simulink model "WorkstationModel"  (Simulink 7.9)
settings: Solver=VariableStepDiscrete  StartTime=0.0  StopTime=100.0  RelTol=1e-3
undefined symbols (not defined in the file or in its folder): des, gcbh
settings Model: Creator=tsprock3  LastModifiedBy=tsprock3
settings DebuggingCC: SimStateOlderReleaseMsg=warning

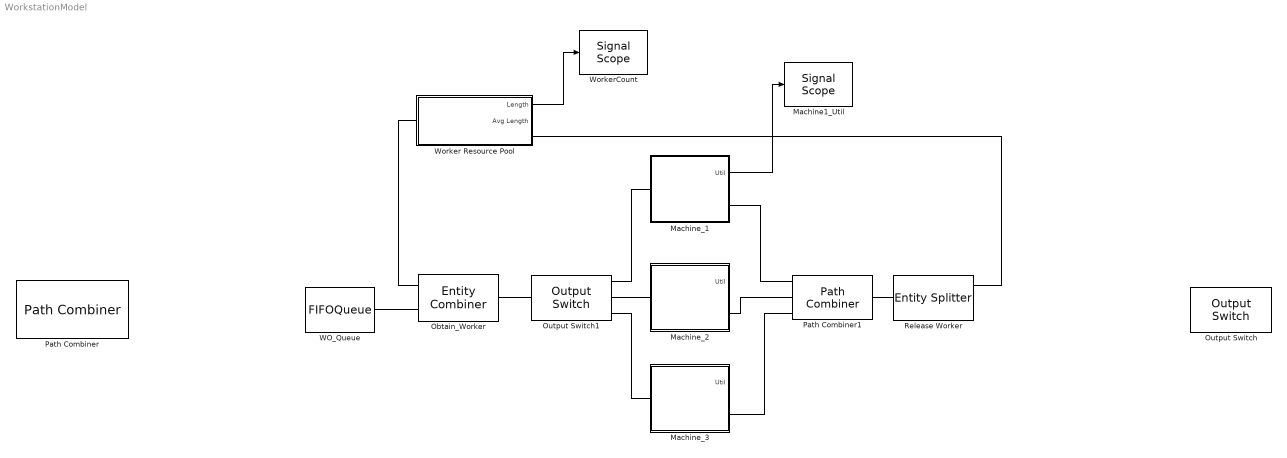
== system WorkstationModel ==
  Machine1_Util : SignalScope  LoadFcn=des.scope.CallbackSupport('seLoadFcn',gcbh)  StartFcn=des.scope.CallbackSupport('seStartFcn',gcbh)  StopFcn=des.scope.CallbackSupport('seStopFcn',gcbh)
      settings: CopyFcn=des.scope.CallbackSupport('seCopyFcn',gcbh)  DeleteFcn=des.scope.CallbackSupport('seDeleteFcn',gcbh)  PreSaveFcn=des.scope.CallbackSupport('sePreSaveFcn',gcbh)  NameChangeFcn=des.scope.CallbackSupport('seNameChangeFcn',gcbh)  OpenFcn=des.scope.CallbackSupport('seOpenFcn',gcbh)
  Machine_1 : Subsystem  mask{mttf=25, mttr=5, ct=3}
      mask prompts: mttf "MTTF (exp)"; mttr "MTTR (exp)"; ct "Process_Time (exp)"
  Machine_2 : Subsystem  mask{mttf=25, mttr=5, ct=3}
      mask prompts: mttf "MTTF (exp)"; mttr "MTTR (exp)"; ct "Process_Time (exp)"
  Machine_3 : Subsystem  mask{mttf=25, mttr=5, ct=3}
      mask prompts: mttf "MTTF (exp)"; mttr "MTTR (exp)"; ct "Process_Time (exp)"
  Obtain_Worker : EntityCombiner  NumberInputPorts=2
  Output Switch : OutputSwitch
  Output Switch1 : OutputSwitch
  Path Combiner : PathCombiner
  Path Combiner1 : PathCombiner
  Release Worker : EntitySplitter  NumberOutputPorts=2
  WO_Queue : FIFOQueue
  Worker Resource Pool : Subsystem  mask{NumberOfEventsPerPeriod=2}
      mask prompts: NumberOfEventsPerPeriod "# of Workers"
  WorkerCount : SignalScope  LoadFcn=des.scope.CallbackSupport('seLoadFcn',gcbh)  StartFcn=des.scope.CallbackSupport('seStartFcn',gcbh)  StopFcn=des.scope.CallbackSupport('seStopFcn',gcbh)
      settings: CopyFcn=des.scope.CallbackSupport('seCopyFcn',gcbh)  DeleteFcn=des.scope.CallbackSupport('seDeleteFcn',gcbh)  PreSaveFcn=des.scope.CallbackSupport('sePreSaveFcn',gcbh)  NameChangeFcn=des.scope.CallbackSupport('seNameChangeFcn',gcbh)  OpenFcn=des.scope.CallbackSupport('seOpenFcn',gcbh)
  wires:
  Worker Resource Pool/1(Length) -> WorkerCount/1
  Machine_1/1(Util) -> Machine1_Util/1
  connections:
  WO_Queue/RConn1 -- Obtain_Worker/LConn2
  Worker Resource Pool/LConn1 -- Obtain_Worker/LConn1
  Obtain_Worker/RConn1 -- Output Switch1/LConn1
  Output Switch1/RConn1 -- Machine_1/LConn1
  Output Switch1/RConn2 -- Machine_2/LConn1
  Output Switch1/RConn3 -- Machine_3/LConn1
  Machine_2/RConn1 -- Path Combiner1/LConn2
  Machine_1/RConn1 -- Path Combiner1/LConn1
  Machine_3/RConn1 -- Path Combiner1/LConn3
  Path Combiner1/RConn1 -- Release Worker/LConn1
  Release Worker/RConn1 -- Worker Resource Pool/RConn1

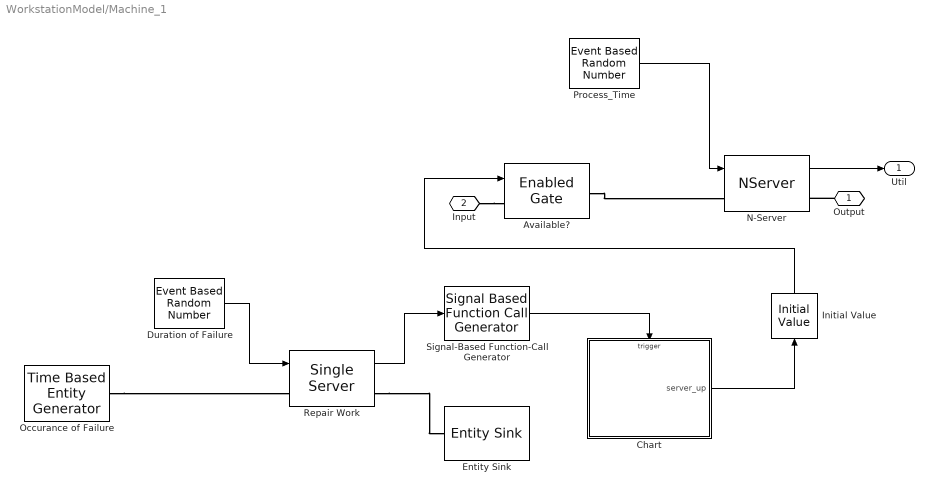
== system WorkstationModel/Machine_1 ==
  Available? : EnabledGate
  Chart : Stateflow chart  TreatAsAtomicUnit=on
  Duration of Failure : EventBasedRandomNumber  meanExp=mttr  meanNorm=5  stdNorm=2  Seed=45272
  Entity Sink : EntitySink
  Initial Value : InitialValue
  N-Server : NServer  NumberOfServers=1  ServiceTimeFrom=Signal port t  StatUtilization=on
      settings: OutputPortMap=o5
  Occurance of Failure : TimeBasedEntityGenerator  Distribution=Exponential  InitialSeed=54923  Mean=mttf  GenerateEntityAtSimulationStart=off  ResponseWhenUnblocked=Delayed restart
  Process_Time : EventBasedRandomNumber  meanExp=ct  Seed=27991
  Repair Work : SingleServer  ServiceTimeFrom=Signal port t  StatNumberInBlock=on
      settings: OutputPortMap=o1
  Signal-Based Function-Call Generator : SignalBasedFunctionCallGenerator  SignalEdgeOption=Either
      settings: InputPortMap=u1
  Output : PMIOPort  Port=1  Side=Right
  Input : PMIOPort  Port=2  Side=Left
  Util : Outport
  wires:
  Initial Value/1 -> Available?/1
  Chart/1(server_up) -> Initial Value/1
  Signal-Based Function-Call Generator/1 -> Chart/Trigger
  Repair Work/1 -> Signal-Based Function-Call Generator/1
  Duration of Failure/1 -> Repair Work/1
  N-Server/1 -> Util/1
  Process_Time/1 -> N-Server/1
  connections:
  Available?/RConn1 -- N-Server/LConn1
  Repair Work/RConn1 -- Entity Sink/LConn1
  Occurance of Failure/RConn1 -- Repair Work/LConn1
  Output/RConn1 -- N-Server/RConn1
  Input/RConn1 -- Available?/LConn1

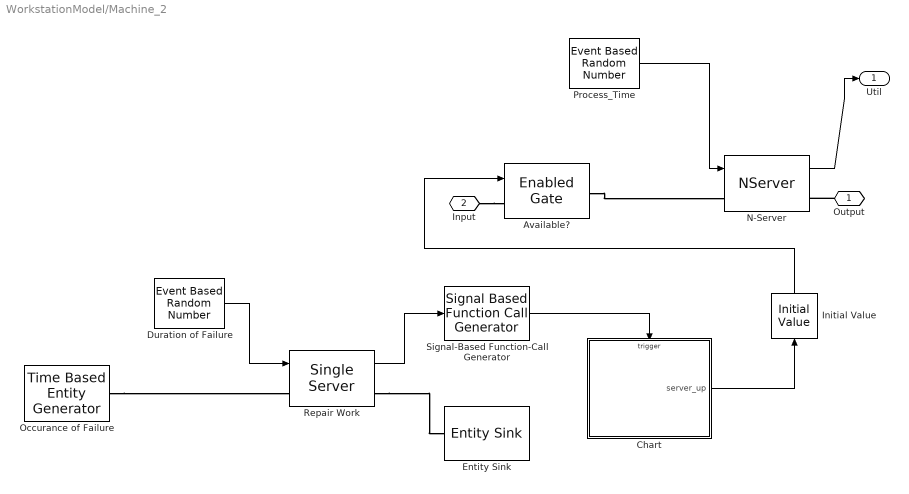
== system WorkstationModel/Machine_2 ==
  Available? : EnabledGate
  Chart : Stateflow chart  TreatAsAtomicUnit=on
  Duration of Failure : EventBasedRandomNumber  meanExp=mttr  meanNorm=5  stdNorm=2  Seed=45272
  Entity Sink : EntitySink
  Initial Value : InitialValue
  N-Server : NServer  NumberOfServers=1  ServiceTimeFrom=Signal port t  StatUtilization=on
      settings: OutputPortMap=o5
  Occurance of Failure : TimeBasedEntityGenerator  Distribution=Exponential  InitialSeed=54923  Mean=mttf  GenerateEntityAtSimulationStart=off  ResponseWhenUnblocked=Delayed restart
  Process_Time : EventBasedRandomNumber  meanExp=ct  Seed=27991
  Repair Work : SingleServer  ServiceTimeFrom=Signal port t  StatNumberInBlock=on
      settings: OutputPortMap=o1
  Signal-Based Function-Call Generator : SignalBasedFunctionCallGenerator  SignalEdgeOption=Either
      settings: InputPortMap=u1
  Output : PMIOPort  Port=1  Side=Right
  Input : PMIOPort  Port=2  Side=Left
  Util : Outport
  wires:
  Initial Value/1 -> Available?/1
  Chart/1(server_up) -> Initial Value/1
  Signal-Based Function-Call Generator/1 -> Chart/Trigger
  Repair Work/1 -> Signal-Based Function-Call Generator/1
  Duration of Failure/1 -> Repair Work/1
  N-Server/1 -> Util/1
  Process_Time/1 -> N-Server/1
  connections:
  Available?/RConn1 -- N-Server/LConn1
  Repair Work/RConn1 -- Entity Sink/LConn1
  Occurance of Failure/RConn1 -- Repair Work/LConn1
  Output/RConn1 -- N-Server/RConn1
  Input/RConn1 -- Available?/LConn1

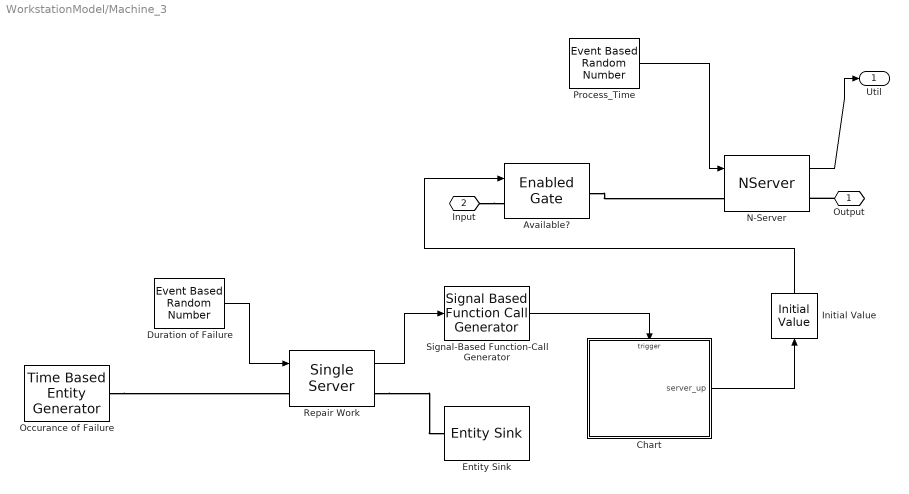
== system WorkstationModel/Machine_3 ==
  Available? : EnabledGate
  Chart : Stateflow chart  TreatAsAtomicUnit=on
  Duration of Failure : EventBasedRandomNumber  meanExp=mttr  meanNorm=5  stdNorm=2  Seed=45272
  Entity Sink : EntitySink
  Initial Value : InitialValue
  N-Server : NServer  NumberOfServers=1  ServiceTimeFrom=Signal port t  StatUtilization=on
      settings: OutputPortMap=o5
  Occurance of Failure : TimeBasedEntityGenerator  Distribution=Exponential  InitialSeed=54923  Mean=mttf  GenerateEntityAtSimulationStart=off  ResponseWhenUnblocked=Delayed restart
  Process_Time : EventBasedRandomNumber  meanExp=ct  Seed=27991
  Repair Work : SingleServer  ServiceTimeFrom=Signal port t  StatNumberInBlock=on
      settings: OutputPortMap=o1
  Signal-Based Function-Call Generator : SignalBasedFunctionCallGenerator  SignalEdgeOption=Either
      settings: InputPortMap=u1
  Output : PMIOPort  Port=1  Side=Right
  Input : PMIOPort  Port=2  Side=Left
  Util : Outport
  wires:
  Initial Value/1 -> Available?/1
  Chart/1(server_up) -> Initial Value/1
  Signal-Based Function-Call Generator/1 -> Chart/Trigger
  Repair Work/1 -> Signal-Based Function-Call Generator/1
  Duration of Failure/1 -> Repair Work/1
  N-Server/1 -> Util/1
  Process_Time/1 -> N-Server/1
  connections:
  Available?/RConn1 -- N-Server/LConn1
  Repair Work/RConn1 -- Entity Sink/LConn1
  Occurance of Failure/RConn1 -- Repair Work/LConn1
  Output/RConn1 -- N-Server/RConn1
  Input/RConn1 -- Available?/LConn1

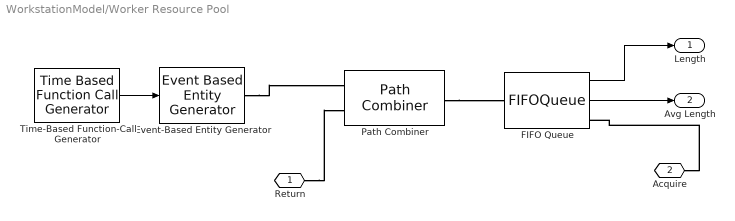
== system WorkstationModel/Worker Resource Pool ==
  Event-Based Entity Generator : EventBasedEntityGenerator  GenerateEntitiesUpon=Function call from port fcn
  FIFO Queue : FIFOQueue  Capacity=5  StatNumberInBlock=on  StatAverageQueueLength=on
      settings: OutputPortMap=o1,o3
  Path Combiner : PathCombiner  NumberInputPorts=2
  Time-Based Function-Call Generator : TimeBasedFunctionCallGenerator  EventGenerationMode=Only at simulation start  NumberOfEventsPerPeriod=NumberOfEventsPerPeriod
  Return : PMIOPort  Port=1  Side=Right
  Acquire : PMIOPort  Port=2  Side=Left
  Length : Outport
  Avg Length : Outport  Port=2
  wires:
  Time-Based Function-Call Generator/1 -> Event-Based Entity Generator/1
  FIFO Queue/2 -> Avg Length/1
  FIFO Queue/1 -> Length/1
  connections:
  Event-Based Entity Generator/RConn1 -- Path Combiner/LConn1
  Path Combiner/RConn1 -- FIFO Queue/LConn1
  Return/RConn1 -- Path Combiner/LConn2
  Acquire/RConn1 -- FIFO Queue/RConn1

== stateflow chart Machine_2/Chart ==
  state Down
    en: server_up = 0;
  state Up
    en: server_up = 1;
  (default) -> Down
  Down -> Up : event
  Up -> Down : event
  data: server_up output double
  events: event input FUNCTION_CALL_EVENT

== stateflow chart Machine_3/Chart ==
  state Down
    en: server_up = 0;
  state Up
    en: server_up = 1;
  (default) -> Down
  Down -> Up : event
  Up -> Down : event
  data: server_up output double
  events: event input FUNCTION_CALL_EVENT

== stateflow chart Machine_1/Chart ==
  state Down
    en: server_up = 0;
  state Up
    en: server_up = 1;
  (default) -> Down
  Down -> Up : event
  Up -> Down : event
  data: server_up output double
  events: event input FUNCTION_CALL_EVENT
